simulink model "T2CDMA"  (Simulink 6.0)
settings: Solver=ode45  StartTime=0.0  StopTime=10.0  RelTol=1e-3
libraries: commseqgen2 x4, commrandsrc2 x2
settings Model: LastModifiedBy=xxgcxy602

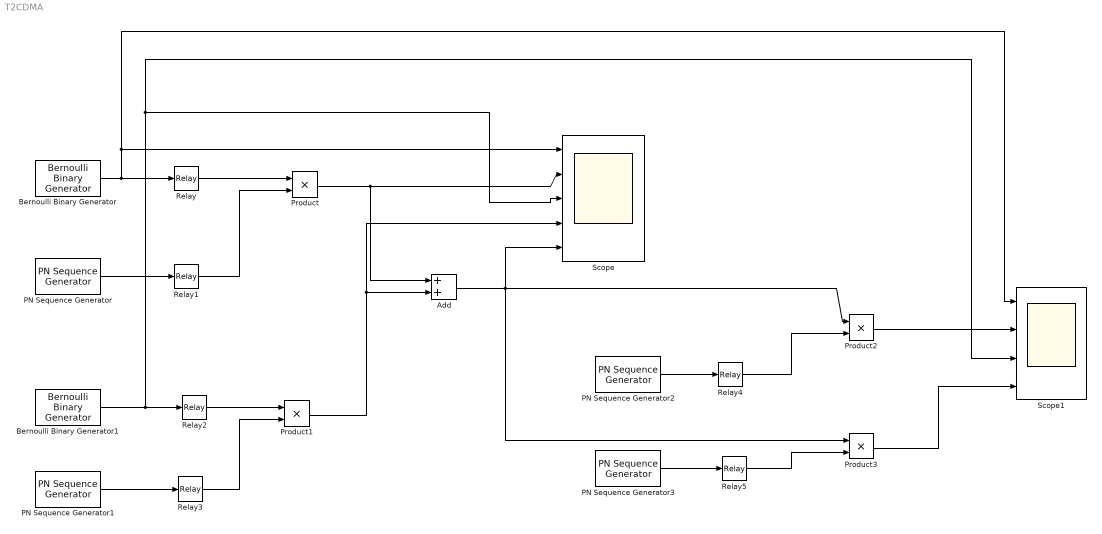
== system T2CDMA ==
  Add : Sum  OutScaling=2^-10
  Bernoulli Binary Generator : commrandsrc2/Bernoulli Binary Generator  P=0.5  seed=61  Ts=1  frameBased=off  sampPerFrame=1  orient=off
  Bernoulli Binary Generator1 : commrandsrc2/Bernoulli Binary Generator  P=0.5  seed=62  Ts=1  frameBased=off  sampPerFrame=1  orient=off
  PN Sequence Generator : commseqgen2/PN Sequence Generator  poly=[1 0 1 1]  ini_sta=[1 0 0]  shift=0  Ts=1/7  frameBased=off  sampPerFrame=1  reset=off
  PN Sequence Generator1 : commseqgen2/PN Sequence Generator  poly=[1 1 0 1]  ini_sta=[1 0 0]  shift=0  Ts=1/7  frameBased=off  sampPerFrame=1  reset=off
  PN Sequence Generator2 : commseqgen2/PN Sequence Generator  poly=[1 0 1 1]  ini_sta=[1 0 0]  shift=0  Ts=1/7  frameBased=off  sampPerFrame=1  reset=off
  PN Sequence Generator3 : commseqgen2/PN Sequence Generator  poly=[1 1 0 1]  ini_sta=[1 0 0]  shift=0  Ts=1/7  frameBased=off  sampPerFrame=1  reset=off
  Product{,1..3} (4 alike) : Product  RndMeth=Zero
  Relay{,1..5} (6 alike) : Relay  OffOutputValue=-1
  Scope : Scope  NumInputPorts=5
      settings: TimeRange=10  YMin=0~-1~0~-1~-2  YMax=1~1~1~1~2
  Scope1 : Scope  NumInputPorts=4
      settings: TimeRange=10  YMin=0~-2~0~-2  YMax=1~2~1~2
  wires:
  Bernoulli Binary Generator/1 -> Relay/1, Scope1/1, Scope/1
  PN Sequence Generator/1 -> Relay1/1
  Bernoulli Binary Generator1/1 -> Relay2/1, Scope1/3, Scope/3
  PN Sequence Generator1/1 -> Relay3/1
  Relay/1 -> Product/1
  Relay1/1 -> Product/2
  Relay2/1 -> Product1/1
  Relay3/1 -> Product1/2
  Product/1 -> Add/1, Scope/2
  Product1/1 -> Add/2, Scope/4
  PN Sequence Generator2/1 -> Relay4/1
  PN Sequence Generator3/1 -> Relay5/1
  Relay5/1 -> Product3/2
  Relay4/1 -> Product2/2
  Add/1 -> Product2/1, Product3/1, Scope/5
  Product3/1 -> Scope1/4
  Product2/1 -> Scope1/2
